simulink model "sys3"  (R2021a)
settings: Solver=VariableStepAuto  StartTime=0.0  StopTime=150  RelTol=1e-3
settings Model: Creator=guilh  LastModifiedBy=guilh

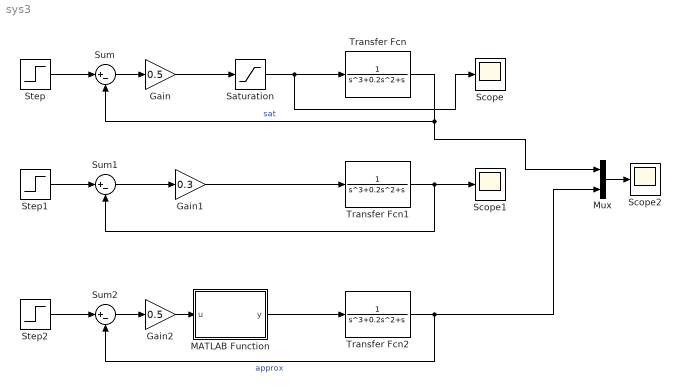
== system sys3 ==
  Gain : Gain  Gain=0.5
  Gain1 : Gain  Gain=0.3
  Gain2 : Gain  Gain=0.5
  MATLAB Function : MATLAB Function  TreatAsAtomicUnit=on
  Mux : Mux  Inputs=2
  Saturation : Saturate  UpperLimit=0.1  LowerLimit=-0.1
  Scope : Scope
  Scope1 : Scope
  Scope2 : Scope
  Step : Step  Time=0  SampleTime=0.1
  Step1 : Step  Time=0  SampleTime=0.1
  Step2 : Step  Time=0  SampleTime=0.1
  Sum : Sum  Inputs=|+-
  Sum1 : Sum  Inputs=|+-
  Sum2 : Sum  Inputs=|+-
  Transfer Fcn : TransferFcn  Denominator=[1 0.2 1 0]
  Transfer Fcn1 : TransferFcn  Denominator=[1 0.2 1 0]
  Transfer Fcn2 : TransferFcn  Denominator=[1 0.2 1 0]
  wires:
  Saturation/1 -> Scope/1, Transfer Fcn/1
  Gain/1 -> Saturation/1
  Step/1 -> Sum/1
  Sum/1 -> Gain/1
  Transfer Fcn/1 -> Mux/1, Sum/2  "sat"
  Gain1/1 -> Transfer Fcn1/1
  Sum1/1 -> Gain1/1
  Step1/1 -> Sum1/1
  Transfer Fcn1/1 -> Sum1/2, Scope1/1
  Transfer Fcn2/1 -> Mux/2, Sum2/2  "approx"
  Sum2/1 -> Gain2/1
  Step2/1 -> Sum2/1
  MATLAB Function/1(y) -> Transfer Fcn2/1
  Gain2/1 -> MATLAB Function/1(u)
  Mux/1 -> Scope2/1

== matlab function sys3/MATLAB Function ==
  data: u input; y output
function y = fcn(u)
    
y = tanh(u/0.05)/10;
